simulink model "L21PendCartsim"  (R2021b)
settings: Solver=FixedStepAuto  StartTime=0.0  StopTime=30  FixedStep=0.001  RelTol=1e-3
InitFcn:
  | L21pendcartparameters;
values from neighbouring files (symbols this model uses):
  A = [0 1 0 0; 0 -d/M m*g/M 0; 0 0 0 1; 0 d/(M*L) -(m+M)*g/(M*L) 0]    [L21pendcartparameters.m]
  B = [0 ; 1/M ; 0 ; -1/(M*L)]    [L21pendcartparameters.m]
  Baug = [B G]    [L21pendcartparameters.m]
  C = [1 0 0 0]    [L21pendcartparameters.m]
  x0 = [0; 0; 0; 0]    [L21pendcartparameters.m]
  xhat0 = [0;0;0;0]    [L21pendcartparameters.m]
undefined symbols (not defined in the file or in its folder): LKB
libraries: simulink x2
settings Model: Creator=vcichella  LastModifiedBy=vcichella_l
settings SolverCC: AlgebraicLoopSolver=TrustRegion
settings DebuggingCC: SFMachineParentedDataDiag=warning

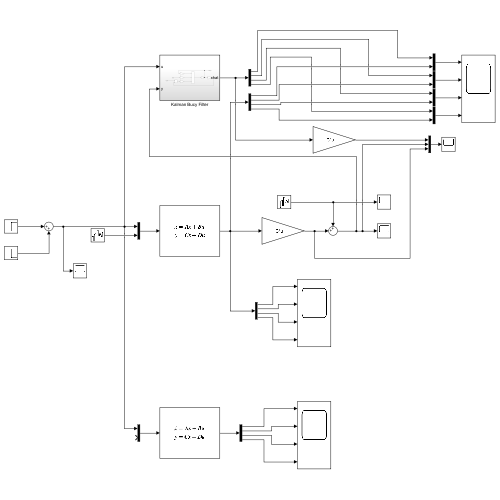
[thumbnail: Simulink's stored preview of the top-level diagram]
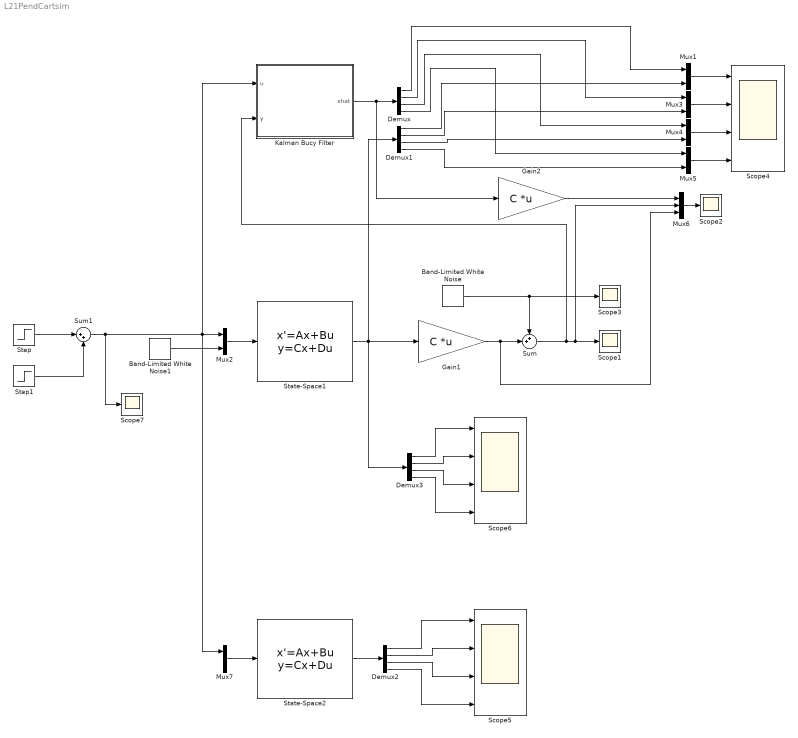
== system L21PendCartsim ==
  Band-Limited White Noise : simulink/Sources/Band-Limited White Noise  Cov=[0.01]  Ts=0.01  seed=[23341]
  Band-Limited White Noise1 : simulink/Sources/Band-Limited White Noise  Cov=[0.0001]  Ts=0.01  seed=[23341]
  Demux{,1..3} (4 alike) : Demux
  Gain1 : Gain  Gain=C  Multiplication=Matrix(K*u)
  Gain2 : Gain  Gain=C  Multiplication=Matrix(K*u)
  Kalman Bucy Filter : Subsystem
  Mux{1..5,7} (6 alike) : Mux  Inputs=2
  Mux6 : Mux  Inputs=3
  Scope{1..3,7} (4 alike) : Scope
  Scope4 : Scope  NumInputPorts=4
  Scope5 : Scope  NumInputPorts=4
  Scope6 : Scope  NumInputPorts=4
  State-Space1 : StateSpace  A=A  B=Baug  C=eye(size(A))  D=zeros(4,2)  InitialCondition=x0
  State-Space2 : StateSpace  A=A  B=Baug  C=eye(size(A))  D=zeros(4,2)  InitialCondition=x0
  Step : Step  Time=5  After=10  SampleTime=0
  Step1 : Step  Time=7  After=-10  SampleTime=0
  Sum : Sum  Inputs=++|
  Sum1 : Sum  Inputs=|++
  wires:
  State-Space1/1 -> Demux3/1, Demux1/1, Gain1/1
  Sum/1 -> Kalman Bucy Filter/2(y), Mux6/2, Scope1/1
  Gain1/1 -> Mux6/3, Sum/2
  Band-Limited White Noise/1 -> Sum/1, Scope3/1
  Kalman Bucy Filter/1(xhat) -> Gain2/1, Demux/1
  Mux1/1 -> Scope4/1
  Mux3/1 -> Scope4/2
  Mux4/1 -> Scope4/3
  Mux5/1 -> Scope4/4
  Demux/1 -> Mux1/1
  Demux1/1 -> Mux1/2
  Demux/2 -> Mux3/1
  Demux1/2 -> Mux3/2
  Demux/3 -> Mux4/1
  Demux1/3 -> Mux4/2
  Demux/4 -> Mux5/1
  Demux1/4 -> Mux5/2
  Mux2/1 -> State-Space1/1
  Sum1/1 -> Scope7/1, Mux7/1, Kalman Bucy Filter/1(u), Mux2/1
  Band-Limited White Noise1/1 -> Mux2/2
  Mux6/1 -> Scope2/1
  Gain2/1 -> Mux6/1
  Mux7/1 -> State-Space2/1
  State-Space2/1 -> Demux2/1
  Demux2/2 -> Scope5/2
  Demux2/3 -> Scope5/3
  Demux2/1 -> Scope5/1
  Demux2/4 -> Scope5/4
  Step/1 -> Sum1/1
  Step1/1 -> Sum1/2
  Demux3/2 -> Scope6/2
  Demux3/3 -> Scope6/3
  Demux3/1 -> Scope6/1
  Demux3/4 -> Scope6/4

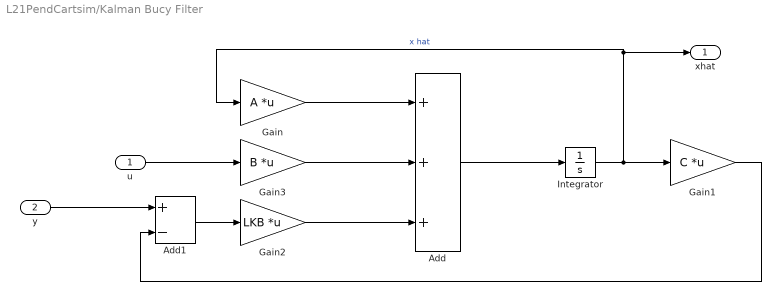
== system L21PendCartsim/Kalman Bucy Filter ==
  u : Inport
  y : Inport  Port=2
  Add : Sum  Inputs=+++
  Add1 : Sum  Inputs=+-
  Gain : Gain  Gain=A  Multiplication=Matrix(K*u)
  Gain1 : Gain  Gain=C  Multiplication=Matrix(K*u)
  Gain2 : Gain  Gain=LKB  Multiplication=Matrix(K*u)
  Gain3 : Gain  Gain=B  Multiplication=Matrix(K*u)
  Integrator : Integrator  InitialCondition=xhat0
  xhat : Outport
  wires:
  Gain3/1 -> Add/2
  u/1 -> Gain3/1
  Gain2/1 -> Add/3
  y/1 -> Add1/1
  Add1/1 -> Gain2/1
  Gain1/1 -> Add1/2
  Gain/1 -> Add/1
  Add/1 -> Integrator/1
  Integrator/1 -> Gain1/1, Gain/1, xhat/1  "x hat"
